simulink model "Lab3"  (R2017a)
settings: Solver=ode3  StartTime=0.0  StopTime=0.008  FixedStep=2e-6  RelTol=1e-5  EnableMultiTasking=on
libraries: commfilt2 x2, commchan3 x1, commsink2 x1, commrandsrc2 x1
settings Model: Creator=Dennis Silage  LastModifiedBy=chris
settings DataIOCC: LimitDataPoints=on  SaveFormat=Array  SignalLoggingSaveFormat=ModelDataLogs
settings OptimizationCC: ExpressionDepthLimit=2147483647  InitFltsAndDblsToZero=on  LifeSpan=inf
settings DebuggingCC: UnderspecifiedInitializationDetection=Classic  MergeDetectMultiDrivingBlocksExec=none  FcnCallInpInsideContextMsg=warning  StateNameClashWarn=warning  SFUnexpectedBacktrackingDiag=warning  SFNoUnconditionalDefaultTransitionDiag=warning  SFExecutionAtInitializationDiag=none
settings HardwareCC: ProdBitPerPointer=32  ProdBitPerSizeT=32  ProdBitPerPtrDiffT=32  ProdLargestAtomicFloat=None  ProdIntDivRoundTo=Undefined  ProdEndianess=Unspecified  ProdWordSize=32  ProdHWDeviceType=32-bit Generic
settings ModelReferenceCC: PropagateSignalLabelsOutOfModel=off
settings GRTTargetCC: TargetLangStandard=C89/C90 (ANSI)  GeneratePreprocessorConditionals=Disable all  CombineOutputUpdateFcns=off  GRTInterface=on
settings ConfigComp: CovMetricSettings=dw  CovHtmlReporting=on  CovSaveCumulativeToWorkspaceVar=on  CovSaveSingleToWorkspaceVar=on  CovExternalEMLEnable=off  CovSFcnEnable=off

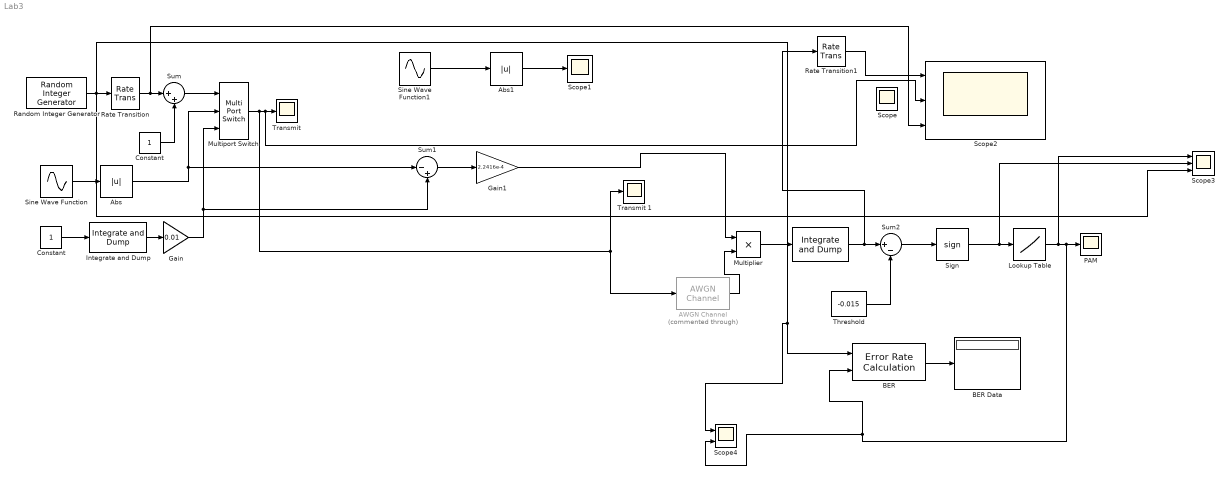
== system Lab3 ==
  " " : commfilt2/Integrate and Dump  obssamples=200  offsetsamples=0  nodump=off  roundingMode=Floor  overflowMode=off  outputDataTypeStr=Inherit: Same as accumulator  outputLastDataTypeStr=Inherit: Same as accumulator
      settings: SourceProductName=Communications System Toolbox
  AWGN Channel : commchan3/AWGN Channel  Commented=through  InputProcessing=Inherited (this choice will be removed - see release notes)  seed=randseed  noiseMode=Variance from mask  EbNodB=40  EsNodB=10  SNRdB=10  bitsPerSym=1  Ps=25  Tsym=400e-6  variance=0
  Abs : Abs
  Abs1 : Abs
  BER : commsink2/Error Rate Calculation  N=2  st_delay=0  cp_mode=Entire frame  subframe=[]  PMode=Port  WsName=ErrorVec  RsMode2=off  stop=off  numErr=100  maxBits=1e6
  BER Data : Display
  Constant : Constant
  "Constant " : Constant  SampleTime=2e-6
  Gain : Gain  Gain=0.01
  Gain1 : Gain  Gain=2.2416e-4
  Integrate and Dump : commfilt2/Integrate and Dump  obssamples=200  offsetsamples=0  nodump=on  roundingMode=Floor  overflowMode=off  outputDataTypeStr=Inherit: Same as accumulator  outputLastDataTypeStr=Inherit: Same as accumulator
      settings: SourceProductName=Communications System Toolbox
  Lookup Table : Lookup_n-D  NumberOfTableDimensions=1  BreakpointsForDimension1=[-1, 1]  Table=[0, 1]  InternalRulePriority=Speed  RndMeth=Nearest  InputSameDT=on
  Multiplier : Product  RndMeth=Zero
  Multiport Switch : MultiPortSwitch  Inputs=2
  "PAM " : Scope
  Random Integer Generator : commrandsrc2/Random Integer Generator  mul=2  seed=randseed  Ts=400e-6  frameBased=off  sampPerFrame=50  orient=on  outDataType=double
  Rate Transition : RateTransition
  Rate Transition1 : RateTransition
  Scope : Scope  NumInputPorts=2
  Scope1 : Scope
  Scope2 : Scope  NumInputPorts=3
  Scope3 : Scope  NumInputPorts=3
  Scope4 : Scope  NumInputPorts=2
  Sign : Signum
  Sine Wave Function : Sin  SineType=Sample based  Amplitude=2  Frequency=2*pi*0.0005  Samples=400  SampleTime=2e-6
  Sine Wave Function1 : Sin  Amplitude=2  Frequency=2*pi*1250  Samples=400  SampleTime=2e-6
  Sum : Sum  Inputs=|++
  Sum1 : Sum  Inputs=|-+
  Sum2 : Sum  Inputs=|+-
  Threshold : Constant  Value=-0.015
  Transmit : Scope
  Transmit 1 : Scope
  wires:
  Rate Transition/1 -> Scope2/3, Sum/1
  Sum/1 -> Multiport Switch/1
  Constant/1 -> Sum/2
  Integrate and Dump/1 -> Gain/1
  "Constant "/1 -> Integrate and Dump/1
  Sine Wave Function/1 -> Abs/1
  Abs/1 -> Multiport Switch/2, Sum1/1
  Sum1/1 -> Gain1/1
  Gain/1 -> Sum1/2, Multiport Switch/3
  Sine Wave Function1/1 -> Abs1/1
  Abs1/1 -> Scope1/1
  Multiplier/1 -> " "/1
  Multiport Switch/1 -> AWGN Channel/1, Transmit 1/1, Scope2/2, Transmit/1
  AWGN Channel/1 -> Multiplier/2
  BER/1 -> BER Data/1
  Sum2/1 -> Sign/1
  Lookup Table/1 -> Scope3/1, "PAM "/1, Scope4/2, BER/2
  Random Integer Generator/1 -> Scope4/1, BER/1, Scope3/3, Rate Transition/1
  Threshold/1 -> Sum2/2
  " "/1 -> Rate Transition1/1, Sum2/1
  Sign/1 -> Scope3/2, Lookup Table/1
  Gain1/1 -> Multiplier/1
  Rate Transition1/1 -> Scope2/1
